simulink model "partial_delay_prog_blk"  (R2019a)
settings: Solver=VariableStepAuto  StartTime=0.0  StopTime=10.0  RelTol=1e-3
libraries: xbsIndex_r4 x2
settings Model: Creator=mybur  LastModifiedBy=mybur

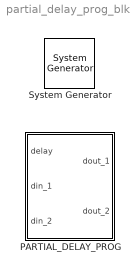
== system partial_delay_prog_blk ==
  " System Generator" : xbsIndex_r4/ System Generator  Tag=genX  xilinxfamily=kintex7  part=xc7k325t  speed=-3  package=fbg676  synthesis_tool=Vivado  clock_wrapper=Clock Enables  directory=./netlist  proj_type=Vivado  Synth_file=Vivado Synthesis Defaults  Impl_file=Vivado Implementation Defaults  testbench=off  simulink_period=1  sysclk_period=10  dcm_input_clock_period=10  incr_netlist=off  trim_vbits=Everywhere in SubSystem  dbl_ovrd=According to Block Masks  core_generation=According to Block Masks  run_coregen=off  deprecated_control=off  eval_field=0  block_type=sysgen
  PARTIAL_DELAY_PROG : Subsystem  mask{async=off, n_ports=2, mux_latency=2}
      mask prompts: async "Asynchronous?"; n_ports "Number of simultaneos ports"; mux_latency "Mux latency"
      mask init:
      | Simulink.Block.eval([gcb, '/partial_delay_prog']);
      | knit_subsystem_to_blackbox('partial_delay_prog');

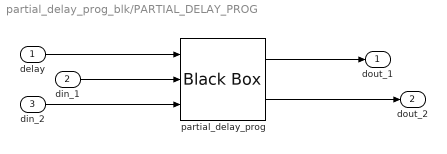
== system partial_delay_prog_blk/PARTIAL_DELAY_PROG ==
  delay : Inport
  din_1 : Inport  Port=2
  din_2 : Inport  Port=3
  partial_delay_prog : xbsIndex_r4/Black Box  init_code=partial_delay_prog_config  sim_method=ISE Simulator  verbose=on  block_type=blackbox2
  dout_1 : Outport
  dout_2 : Outport  Port=2
  wires:
  delay/1 -> partial_delay_prog/1
  din_1/1 -> partial_delay_prog/2
  din_2/1 -> partial_delay_prog/3
  partial_delay_prog/1 -> dout_1/1
  partial_delay_prog/2 -> dout_2/1
